simulink model "configurable_pwm"  (R2014a)
settings: Solver=VariableStepDiscrete  StartTime=0.0  StopTime=100000  RelTol=1e-3
libraries: hdlsllib x4, simulink x2
settings Model: Creator=hirn.j  LastModifiedBy=hirn.j
settings OptimizationCC: BlockReduction=off  ConditionallyExecuteInputs=off  InlineParams=on
settings DebuggingCC: AlgebraicLoopMsg=error
settings HardwareCC: ProdHWDeviceType=ASIC/FPGA->ASIC/FPGA  ProdEqTarget=off

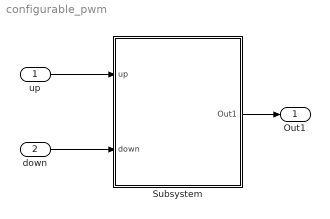
== system configurable_pwm ==
  up : Inport  OutDataTypeStr=boolean  SampleTime=1
  down : Inport  Port=2  OutDataTypeStr=boolean  SampleTime=1
  Subsystem : Subsystem  TreatAsAtomicUnit=on  SystemSampleTime=1
  Out1 : Outport  SampleTime=1
  wires:
  up/1 -> Subsystem/1(up)
  down/1 -> Subsystem/2(down)
  Subsystem/1(Out1) -> Out1/1

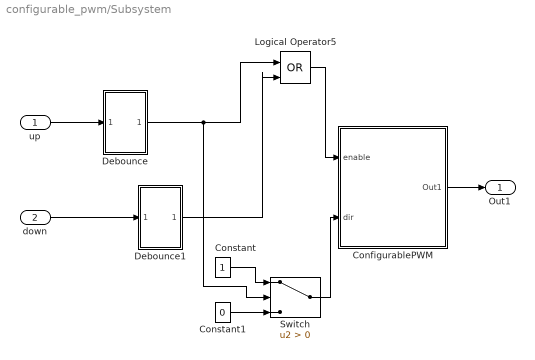
== system configurable_pwm/Subsystem ==
  up : Inport  OutDataTypeStr=boolean  SampleTime=1
  down : Inport  Port=2  OutDataTypeStr=boolean  SampleTime=1
  ConfigurablePWM : Subsystem
  Constant : Constant  OutDataTypeStr=boolean
  Constant1 : Constant  Value=0  OutDataTypeStr=boolean
  Debounce : Subsystem
  Debounce1 : Subsystem
  Logical Operator5 : Logic  Operator=OR  IconShape=distinctive  AllPortsSameDT=off  OutDataTypeStr=boolean  SampleTime=1
  Switch : Switch  Criteria=u2 > Threshold
  Out1 : Outport  SampleTime=1
  wires:
  Debounce/1(Out1) -> Switch/2, Logical Operator5/1
  Logical Operator5/1 -> ConfigurablePWM/1(enable)
  up/1 -> Debounce/1(In1)
  down/1 -> Debounce1/1(In1)
  Constant/1 -> Switch/1
  Switch/1 -> ConfigurablePWM/2(dir)
  Constant1/1 -> Switch/3
  Debounce1/1(Out1) -> Logical Operator5/2
  ConfigurablePWM/1(Out1) -> Out1/1

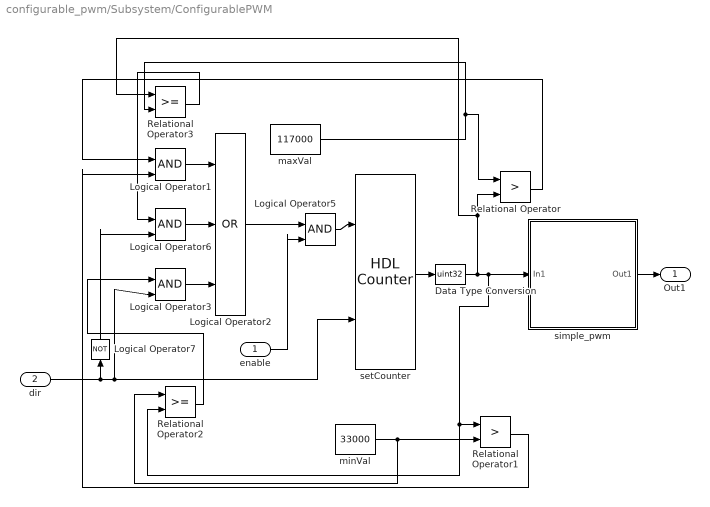
== system configurable_pwm/Subsystem/ConfigurablePWM ==
  enable : Inport  OutDataTypeStr=boolean
  dir : Inport  Port=2  OutDataTypeStr=boolean
  Data Type Conversion : DataTypeConversion  OutDataTypeStr=uint32
  Logical Operator{1,3,5..6} (4 alike) : Logic  IconShape=distinctive  AllPortsSameDT=off  OutDataTypeStr=boolean  SampleTime=1
  Logical Operator2 : Logic  Operator=OR  Inputs=3  IconShape=distinctive  AllPortsSameDT=off  OutDataTypeStr=boolean  SampleTime=1
  Logical Operator7 : Logic  Operator=NOT  IconShape=distinctive  AllPortsSameDT=off  OutDataTypeStr=boolean  SampleTime=1
  Relational Operator : RelationalOperator  Operator=>  OutDataTypeStr=boolean
  Relational Operator1 : RelationalOperator  Operator=>  OutDataTypeStr=boolean
  Relational Operator2 : RelationalOperator  OutDataTypeStr=boolean
  Relational Operator3 : RelationalOperator  OutDataTypeStr=boolean
  maxVal : Constant  Value=117000  OutDataTypeStr=uint32
  minVal : Constant  Value=33000  OutDataTypeStr=uint32
  setCounter : hdlsllib/HDL Operations/HDL Counter  CountType=Count limited  CountInit=75000  CountStep=6000  CountMax=120000  CountFromType=Specify  CountFrom=30000  CountResetPort=off  CountLoadPort=off  CountEnbPort=on  CountDirPort=on  CountDataType=Unsigned  CountWordLen=20  CountFracLen=0  CountSampTime=1
  simple_pwm : Subsystem
  Out1 : Outport
  wires:
  Logical Operator7/1 -> Logical Operator6/2
  enable/1 -> Logical Operator5/2
  dir/1 -> Logical Operator7/1, Logical Operator3/2, setCounter/2
  setCounter/1 -> Data Type Conversion/1
  Logical Operator1/1 -> Logical Operator2/1
  Relational Operator/1 -> Logical Operator1/1
  maxVal/1 -> Relational Operator3/2, Relational Operator/1
  Logical Operator5/1 -> setCounter/1
  Relational Operator1/1 -> Logical Operator1/2
  Logical Operator2/1 -> Logical Operator5/1
  Logical Operator6/1 -> Logical Operator2/2
  Logical Operator3/1 -> Logical Operator2/3
  simple_pwm/1(Out1) -> Out1/1
  Data Type Conversion/1 -> Relational Operator2/2, Relational Operator1/1, simple_pwm/1(In1), Relational Operator3/1, Relational Operator/2
  minVal/1 -> Relational Operator2/1, Relational Operator1/2
  Relational Operator2/1 -> Logical Operator3/1
  Relational Operator3/1 -> Logical Operator6/1

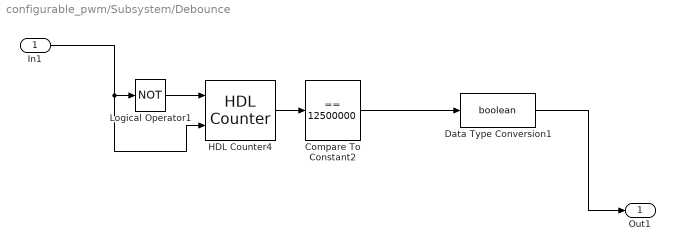
== system configurable_pwm/Subsystem/Debounce ==
  In1 : Inport
  Compare To Constant2 : simulink/Logic and Bit Operations/Compare To Constant  relop===  const=12500000  OutDataTypeStr=boolean
  Data Type Conversion1 : DataTypeConversion  OutDataTypeStr=boolean
  HDL Counter4 : hdlsllib/HDL Operations/HDL Counter  CountType=Free running  CountInit=0  CountStep=1  CountMax=100  CountFromType=Initial value  CountFrom=0  CountResetPort=on  CountLoadPort=off  CountEnbPort=on  CountDirPort=off  CountDataType=Unsigned  CountWordLen=32  CountFracLen=0  CountSampTime=1
  Logical Operator1 : Logic  Operator=NOT  IconShape=distinctive  AllPortsSameDT=off  OutDataTypeStr=boolean  SampleTime=1
  Out1 : Outport
  wires:
  Logical Operator1/1 -> HDL Counter4/1
  Compare To Constant2/1 -> Data Type Conversion1/1
  In1/1 -> HDL Counter4/2, Logical Operator1/1
  Data Type Conversion1/1 -> Out1/1
  HDL Counter4/1 -> Compare To Constant2/1

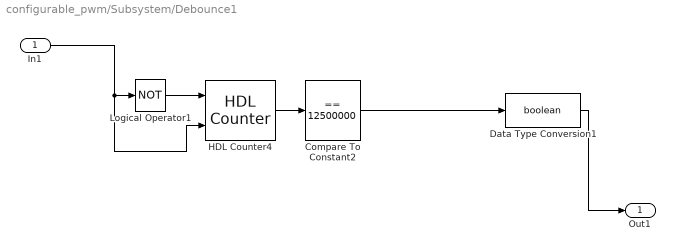
== system configurable_pwm/Subsystem/Debounce1 ==
  In1 : Inport
  Compare To Constant2 : simulink/Logic and Bit Operations/Compare To Constant  relop===  const=12500000  OutDataTypeStr=boolean
  Data Type Conversion1 : DataTypeConversion  OutDataTypeStr=boolean
  HDL Counter4 : hdlsllib/HDL Operations/HDL Counter  CountType=Free running  CountInit=0  CountStep=1  CountMax=100  CountFromType=Initial value  CountFrom=0  CountResetPort=on  CountLoadPort=off  CountEnbPort=on  CountDirPort=off  CountDataType=Unsigned  CountWordLen=32  CountFracLen=0  CountSampTime=1
  Logical Operator1 : Logic  Operator=NOT  IconShape=distinctive  AllPortsSameDT=off  OutDataTypeStr=boolean  SampleTime=1
  Out1 : Outport
  wires:
  Logical Operator1/1 -> HDL Counter4/1
  Compare To Constant2/1 -> Data Type Conversion1/1
  In1/1 -> HDL Counter4/2, Logical Operator1/1
  Data Type Conversion1/1 -> Out1/1
  HDL Counter4/1 -> Compare To Constant2/1

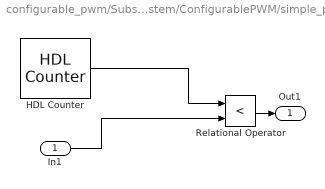
== system configurable_pwm/Subsystem/ConfigurablePWM/simple_pwm ==
  In1 : Inport  OutDataTypeStr=uint32
  HDL Counter : hdlsllib/HDL Operations/HDL Counter  CountType=Count limited  CountInit=0  CountStep=1  CountMax=1000000  CountFromType=Initial value  CountFrom=0  CountResetPort=off  CountLoadPort=off  CountEnbPort=off  CountDirPort=off  CountDataType=Unsigned  CountWordLen=20  CountFracLen=0  CountSampTime=1
  Relational Operator : RelationalOperator  Operator=<  OutDataTypeStr=boolean  SampleTime=1
  Out1 : Outport
  wires:
  Relational Operator/1 -> Out1/1
  HDL Counter/1 -> Relational Operator/1
  In1/1 -> Relational Operator/2
